simulink model "SteadyStateChar"  (R2022b)
settings: Solver=ode45  StartTime=0.0  StopTime=simStopTime  RelTol=1e-3  EnableMultiTasking=on
InitFcn:
  | tmp_stop_time_as_str = get_param(gcs, 'StopTime');
  | tmp_stop_time = str2double(tmp_stop_time_as_str);
  | clear tmp_stop_time_as_str;
StopFcn:
  | clear tmp_stop_time;
  | 
  | save("./dataRepo/" + "logsout_" + string(datetime('now','Format','yyyy-MM-dd_HH_mm_ss'))+".mat", "logsout")
  | 
  | 
  | 
  | tmp_sig_mainOutput = [logsout{1}.Values.Time, logsout{1}.Values.Data];
  | 
  | tmp_sig_1 = interp1( logsout{2}.Values.Time, logsout{2}.Values.Data, tmp_sig_mainOutput(:,1));
  | tmp_sig_2 = interp1( logsout{3}.Values.Time, logsout{3}.Values.Data, tmp_sig_mainOutput(:,1));
  | 
  | tmp_data = [tmp_sig_mainOutput, tmp_sig_1, tmp_sig_2];
  | 
  | writematrix(tmp_data, "./dataRepo/" + "logsout_" + string(datetime('now','Format','yyyy-MM-dd_HH_mm_ss'))+"_processed.csv")
  | 
  | clear tmp_data tmp_sig_mainOutput tmp_sig_1 tmp_sig_2
values from neighbouring files (symbols this model uses):
  simStopTime = steadyTime * rowidx    [measurementSetup.m]
undefined symbols (not defined in the file or in its folder): Advantech, PCI
libraries: sldrtlib x3
settings Model: Creator=Admin  LastModifiedBy=admin
settings SolverCC: AlgebraicLoopSolver=TrustRegion
settings DataIOCC: SaveFormat=Array  SaveOutput=off  DSMLogging=off  SaveTime=off  ReturnWorkspaceOutputs=off
settings OptimizationCC: LifeSpan=inf
settings DebuggingCC: UnconnectedInputMsg=warning  UnconnectedOutputMsg=warning  UnconnectedLineMsg=warning  SFUnexpectedBacktrackingDiag=warning  SFNoUnconditionalDefaultTransitionDiag=warning  SFExecutionAtInitializationDiag=none  SFMachineParentedDataDiag=warning  ArithmeticOperatorsInVariantConditions=warning
settings HardwareCC: ProdBitPerPointer=32  ProdBitPerSizeT=32  ProdBitPerPtrDiffT=32  ProdLargestAtomicFloat=None  ProdIntDivRoundTo=Undefined  ProdEndianess=Unspecified  ProdWordSize=32  ProdHWDeviceType=32-bit Generic
settings ModelReferenceCC: PropagateSignalLabelsOutOfModel=off
settings SFSimCC: SimUseLocalCustomCode=off  CustomCodeUndefinedFunction=UseInterfaceOnly
settings RTWCC: RTWUseLocalCustomCode=off
settings CodeAppCC: StateflowObjectComments=on
settings GRTTargetCC: TargetLangStandard=C89/C90 (ANSI)
settings ConfigComp: CovMetricSettings=dw  CovSaveCumulativeToWorkspaceVar=on  CovSaveSingleToWorkspaceVar=on  CovExternalEMLEnable=off

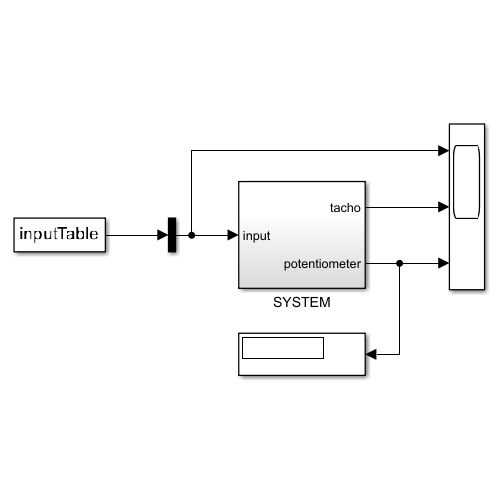
[thumbnail: Simulink's stored preview of the top-level diagram]
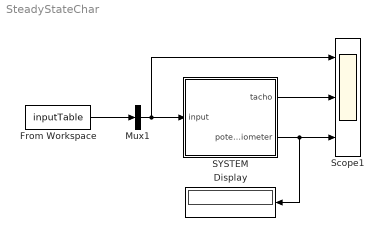
== system SteadyStateChar ==
  Display : Display
  From Workspace : FromWorkspace  VariableName=inputTable  Interpolate=off  OutputAfterFinalValue=Holding final value
  Mux1 : Mux  Inputs=1
  SYSTEM : Subsystem
  Scope1 : Scope  NumInputPorts=3
  wires:
  SYSTEM/2(potentiometer) -> Display/1, Scope1/3
  Mux1/1 -> Scope1/1, SYSTEM/1(input)
  SYSTEM/1(tacho) -> Scope1/2
  From Workspace/1 -> Mux1/1

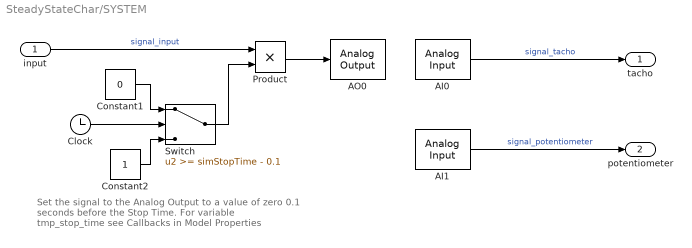
== system SteadyStateChar/SYSTEM ==
  note: Set the signal to the Analog Output to a value of zero
      | 0.1 seconds before the Stop Time.
      |
      | For variable tmp_stop_time see
      | Callbacks in Model Properties
  input : Inport
  AI0 : sldrtlib/Analog Input  SampleTime=0.1  MaxMissedTicks=10  ShowMissedTicks=off  YieldWhenWaiting=off  DrvName=Advantech/PCI-1711  DrvAddress=4294967295  DrvOptions=zeros(1,0)  Channels=1  RangeMode=1  VoltRange=1  DataType=1
      settings: AttributesFormatString=Advantech\nPCI-1711 [auto]
  AI1 : sldrtlib/Analog Input  SampleTime=0.1  MaxMissedTicks=10  ShowMissedTicks=off  YieldWhenWaiting=off  DrvName=Advantech/PCI-1711  DrvAddress=4294967295  DrvOptions=zeros(1,0)  Channels=2  RangeMode=1  VoltRange=1  DataType=1
      settings: AttributesFormatString=Advantech\nPCI-1711 [auto]
  AO0 : sldrtlib/Analog Output  SampleTime=0.1  MaxMissedTicks=10  ShowMissedTicks=off  YieldWhenWaiting=off  DrvName=Advantech/PCI-1711  DrvAddress=4294967295  DrvOptions=zeros(1,0)  Channels=1  RangeMode=1  VoltRange=2  InitialValue=[]  FinalValue=[]
      settings: AttributesFormatString=Advantech\nPCI-1711 [auto]
  Clock : Clock
  Constant1 : Constant  Value=0
  Constant2 : Constant
  Product : Product
  Switch : Switch  Threshold=simStopTime - 0.1  SaturateOnIntegerOverflow=off  InputSameDT=off
  tacho : Outport
  potentiometer : Outport  Port=2
  wires:
  AI0/1 -> tacho/1  "signal_tacho"
  AI1/1 -> potentiometer/1  "signal_potentiometer"
  input/1 -> Product/1  "signal_input"
  Product/1 -> AO0/1
  Constant2/1 -> Switch/3
  Constant1/1 -> Switch/1
  Switch/1 -> Product/2
  Clock/1 -> Switch/2
